simulink model "ADAS_System"  (R2025b)
settings: Solver=VariableStepAuto  StartTime=0.0  StopTime=50  FixedStep=0.1  RelTol=1e-3
values from neighbouring files (symbols this model uses):
  fs = 100    [init_ADAS.m]
  v_ego = 30    [init_ADAS.m]
  v_lead = 25    [init_ADAS.m]
libraries: simulink x2
(part 2 of 2)

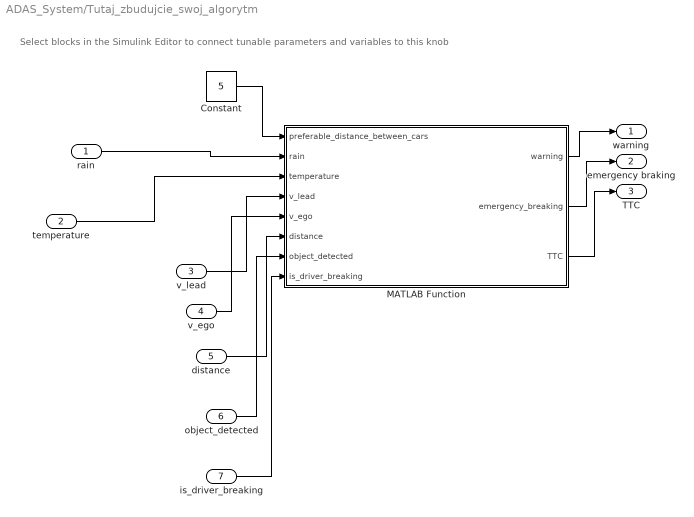
== system ADAS_System/Tutaj_zbudujcie_swoj_algorytm ==
  note: Select blocks in the Simulink Editor to connect tunable parameters and variables to this knob
  rain : Inport
  temperature : Inport  Port=2
  v_lead : Inport  Port=3
  v_ego : Inport  Port=4
  distance : Inport  Port=5
  object_detected : Inport  Port=6
  is_driver_breaking : Inport  Port=7
  Constant : Constant  Value=5
  MATLAB Function : MATLAB Function  TreatAsAtomicUnit=on
  warning : Outport
  emergency braking : Outport  Port=2
  "TTC " : Outport  Port=3
  wires:
  v_lead/1 -> MATLAB Function/4(v_lead)
  v_ego/1 -> MATLAB Function/5(v_ego)
  object_detected/1 -> MATLAB Function/7(object_detected)
  MATLAB Function/1(warning) -> warning/1
  MATLAB Function/3(TTC) -> "TTC "/1
  MATLAB Function/2(emergency_breaking) -> emergency braking/1
  distance/1 -> MATLAB Function/6(distance)
  Constant/1 -> MATLAB Function/1(preferable_distance_between_cars)
  is_driver_breaking/1 -> MATLAB Function/8(is_driver_breaking)
  temperature/1 -> MATLAB Function/3(temperature)
  rain/1 -> MATLAB Function/2(rain)

== matlab function ADAS_System/Tutaj_zbudujcie_swoj_algorytm/MATLAB Function ==
  data: preferable_distance_between_cars input; rain input; temperature input; v_lead input; warning output; v_ego input; distance input; object_detected input; emergency_breaking output; TTC output; is_driver_breaking input
function [warning,emergency_breaking,TTC] = AutonomousEmergencyBraking(preferable_distance_between_cars, rain, temperature, v_lead,v_ego,distance,object_detected, is_driver_breaking)
    if object_detected == false
        warning = 0;
        emergency_breaking = 0;
        TTC = 0;
        return
    end


    mi_rain=0.4;
    mi_snow=0.2;
    mi_normal=0.7;
    g= 9.81;

    s_breaking_rain=(v_ego^2)/(2*mi_rain*g);
    s_breaking_snow=(v_ego^2)/(2*mi_snow*g);
    s_breaking_normal=(v_ego^2)/(2*g*mi_normal*g);


    if rain==0
        preferable_distance_between_cars=preferable_distance_between_cars+ s_breaking_normal;
    else
        if temperature>0
            preferable_distance_between_cars=preferable_distance_between_cars+s_breaking_rain;
        else
            preferable_distance_between_cars=preferable_distance_between_cars+s_breaking_snow;
        end
    end


    breaking_distance = distance - preferable_distance_between_cars;
    v_rel = v_ego - v_lead;
    
    if v_rel <= 0
        TTC = inf;
        TTR = inf;
        TTres = inf;
    else
        TTC = distance / v_rel;
        TTR = breaking_distance / v_rel;
        TTres = v_rel/8;
    end
    FinTres = TTres + 0.7;
    
    if TTR < FinTres
        warning = 1;
        if is_driver_breaking == 0
            emergency_breaking = 1;
        else
            emergency_breaking = 0;
        end
    else
        if TTR < (FinTres + 1.0) && TTR >= FinTres
            warning = 1;
            emergency_breaking = 0;
        else
            warning = 0;
            emergency_breaking = 0;
        end
    end

== matlab function ADAS_System/MATLAB Function ==
  settings: updateMethod=DISCRETE
  data: raw_distance input; clean_distance output; fs input
function clean_distance = radar_filter(raw_distance, fs)
    persistent last_dist;
    
    % Inicjalizacja przy pierwszym kroku symulacji
    if isempty(last_dist)
        last_dist = raw_distance;
    end  
    
    % Obliczenie kroku czasu na podstawie częstotliwości próbkowania
    dt = 1 / fs; 
    
    tau = 0.02; 
    
    % Dynamiczne obliczenie wagi dla nowego pomiaru
    alpha = dt / (tau + dt); 
    
    % Filtracja: waga_nowego * nowy_pomiar + waga_starego * stary_pomiar
    clean_distance = alpha * raw_distance + (1 - alpha) * last_dist;
    
    % Zapisanie obecnej wartości na potrzeby kolejnego kroku
    last_dist = clean_distance;
end
